simulink model "PI_Controller"  (R2020b)
settings: Solver=VariableStepAuto  StartTime=0.0  StopTime=10.0  RelTol=1e-3
model workspace (MAT data in the model file):
  Ki = Simulink.Parameter
  Ki.Value = 40
  Ki.DataType = 'auto'
  Ki.Dimensions = [1 1]
  Kp = Simulink.Parameter
  Kp.Value = 1500
  Kp.DataType = 'auto'
  Kp.Dimensions = [1 1]
settings Model: DataDictionary=Prob3_2005160.sldd  Creator=shoun  LastModifiedBy=shoun

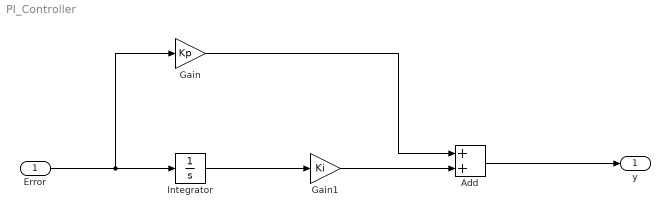
== system PI_Controller ==
  Error : Inport
  Add : Sum
  Gain : Gain  Gain=Kp
  Gain1 : Gain  Gain=Ki
  Integrator : Integrator
  y : Outport
  wires:
  Error/1 -> Gain/1, Integrator/1
  Integrator/1 -> Gain1/1
  Gain1/1 -> Add/2
  Gain/1 -> Add/1
  Add/1 -> y/1
